simulink model "DC_Motor_State_Space"  (R2024b)
settings: Solver=FixedStepAuto  StartTime=0.0  StopTime=10.0  FixedStep=1e-4  RelTol=1e-3
values from neighbouring files (symbols this model uses):
  A = [-R/L -Kb/L 0; Kt/J -B/J 0; 0 1 0]    [Parameters.m]
  B = 15e-6    (= 1.5e-05)    [Parameters.m]
  b = [1/L; 0 ; 0]    [Parameters.m]
  C = [1 0 0; 0 1 0; 0 0 1]    [Parameters.m]
  D = [0 ; 0; 0]    [Parameters.m]
  J = 40e-7    (= 4e-06)    [Parameters.m]
  Kb = 39.3e-3    (= 0.0393)    [Parameters.m]
  Kt = 0.0393    [Parameters.m]
  L = 0.154    [Parameters.m]
  R = 7.94    [Parameters.m]
settings Model: Creator=Nabil  LastModifiedBy=Nabil

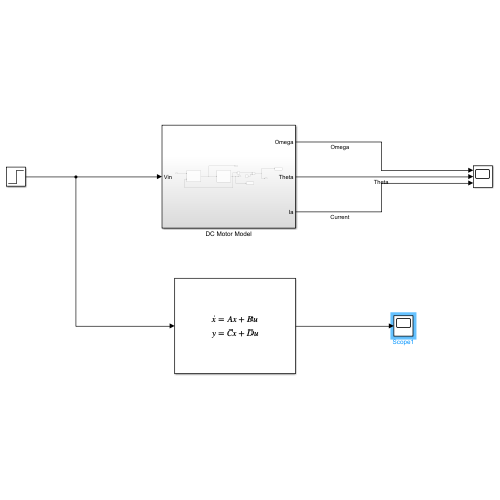
[thumbnail: Simulink's stored preview of the top-level diagram]
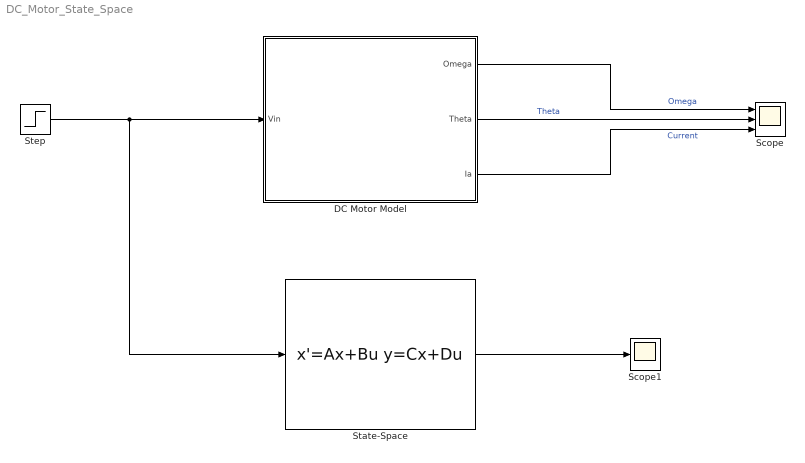
== system DC_Motor_State_Space ==
  DC Motor Model : Subsystem
  Scope : Scope  NumInputPorts=3
  Scope1 : Scope
  State-Space : StateSpace  A=A  B=b  C=C  D=D  InitialCondition=0
  Step : Step  SampleTime=0
  wires:
  Step/1 -> State-Space/1, DC Motor Model/1(Vin)
  DC Motor Model/1(Omega) -> Scope/1  "Omega"
  DC Motor Model/2(Theta) -> Scope/2  "Theta"
  DC Motor Model/3(Ia) -> Scope/3  "Current"
  State-Space/1 -> Scope1/1

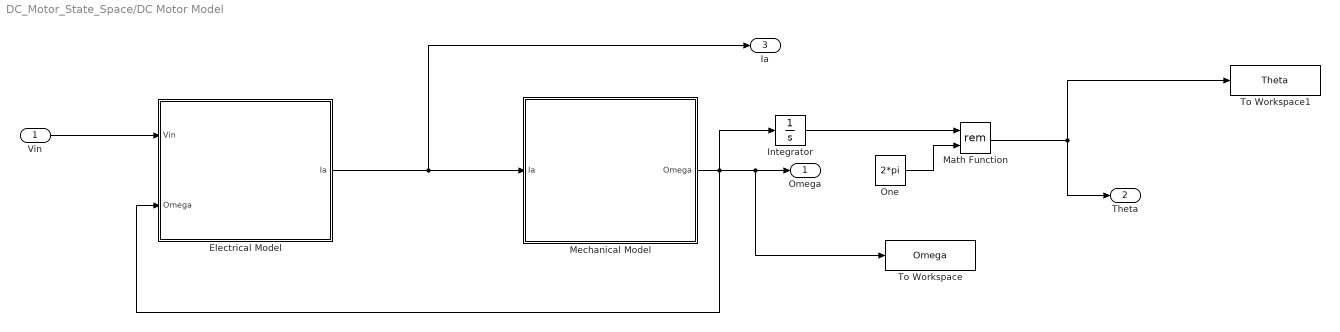
== system DC_Motor_State_Space/DC Motor Model ==
  Vin : Inport
  Electrical Model : Subsystem
  Integrator : Integrator  WrappedStateUpperValue=2*pi  WrappedStateLowerValue=0
  Math Function : Math  Operator=rem
  Mechanical Model : Subsystem
  One : Constant  Value=2*pi  OutDataTypeStr=Inherit: Inherit via back propagation
  To Workspace : ToWorkspace  VariableName=Omega  SaveFormat=Timeseries  SampleTime=-1
  To Workspace1 : ToWorkspace  VariableName=Theta  SaveFormat=Timeseries  SampleTime=-1
  Omega : Outport
  Theta : Outport  Port=2
  Ia : Outport  Port=3
  wires:
  Vin/1 -> Electrical Model/1(Vin)
  Mechanical Model/1(Omega) -> To Workspace/1, Omega/1, Integrator/1, Electrical Model/2(Omega)
  Electrical Model/1(Ia) -> Ia/1, Mechanical Model/1(Ia)
  Integrator/1 -> Math Function/1
  Math Function/1 -> Theta/1, To Workspace1/1
  One/1 -> Math Function/2

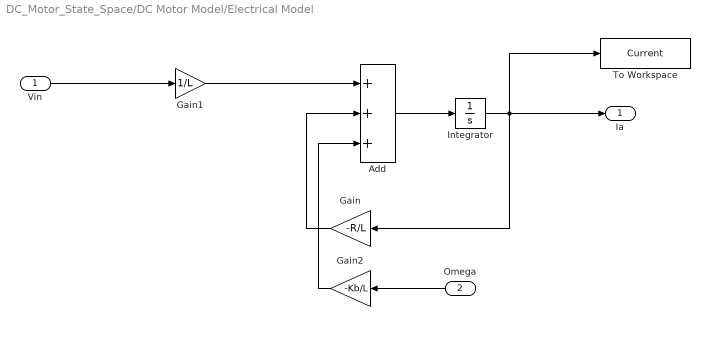
== system DC_Motor_State_Space/DC Motor Model/Electrical Model ==
  Vin : Inport
  Omega : Inport  Port=2
  Add : Sum  Inputs=+++
  Gain : Gain  Gain=-R/L
  Gain1 : Gain  Gain=1/L
  Gain2 : Gain  Gain=-Kb/L
  Integrator : Integrator
  To Workspace : ToWorkspace  VariableName=Current  SaveFormat=Timeseries  SampleTime=-1
  Ia : Outport
  wires:
  Add/1 -> Integrator/1
  Vin/1 -> Gain1/1
  Integrator/1 -> Ia/1, Gain/1, To Workspace/1
  Omega/1 -> Gain2/1
  Gain/1 -> Add/2
  Gain1/1 -> Add/1
  Gain2/1 -> Add/3

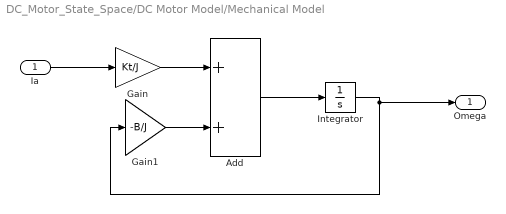
== system DC_Motor_State_Space/DC Motor Model/Mechanical Model ==
  Ia : Inport
  Add : Sum
  Gain : Gain  Gain=Kt/J
  Gain1 : Gain  Gain=-B/J
  Integrator : Integrator
  Omega : Outport
  wires:
  Integrator/1 -> Omega/1, Gain1/1
  Gain1/1 -> Add/2
  Gain/1 -> Add/1
  Ia/1 -> Gain/1
  Add/1 -> Integrator/1
